simulink model "SPHERE_model4_PID_screenshot"  (R2020a)
settings: Solver=ode4  StartTime=0.0  StopTime=100  FixedStep=0.01428571  RelTol=1e-3
values from neighbouring files (symbols this model uses):
  Final_val = 18    [Initial_script.m]    (also in Initial_script_test.m = -28; Initial_script_test2.m = -28)
  K = 25.937    [Initial_script.m]    (also in Initial_script_test.m; Initial_script_test2.m)
  L = -[ M2*l*(-2*l + R) - 2*J2, 0, -2*M2*l*g ]    [Initial_script.m]    (also in Initial_script_test.m; Initial_script_test2.m)
  M = [ J1 + 2*J2 + M1*R^2 + M2*(2*l^2 - 3*R*l + R^2), -Tv, 2*l*g*M2 ]    [Initial_script.m]    (also in Initial_script_test.m; Initial_script_test2.m)
  Smax = 502    [Initial_script.m]    (also in Initial_script_test.m; Initial_script_test2.m)
  Smin = -480    [Initial_script.m]    (also in Initial_script_test.m; Initial_script_test2.m)
  Step_time = 3.18    [Initial_script.m]    (also in Initial_script_test.m = 4.45; Initial_script_test2.m = 4.5)
  Top = 0.015    [Initial_script.m]    (also in Initial_script_test.m; Initial_script_test2.m)
libraries: simulink x2
settings Model: Creator=Adrian  LastModifiedBy=Adrian

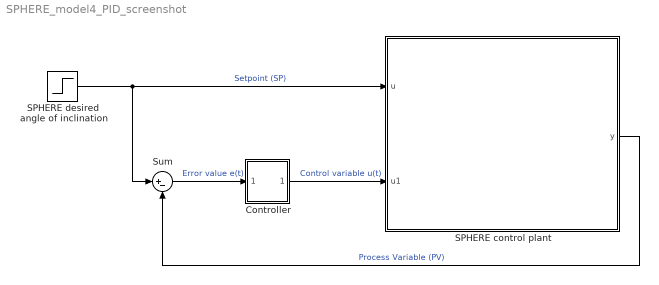
== system SPHERE_model4_PID_screenshot ==
  Controller : Subsystem  mask{Parameter1=}
      mask prompts: Parameter1 "Controller"
  SPHERE control plant : Subsystem
      mask Display: image('C:\Users\Adrian\Documents\Praca Magisterska\Robot kulisty by Adrian\Praca Magisterska\LaTex\Pictures\Old\sphere_full.PNG'); % Use "Edit Image" on toolstrip to change.
  SPHERE desired angle of inclination : Step  Time=Step_time  After=Final_val  SampleTime=0
  Sum : Sum  Inputs=|+-
  wires:
  SPHERE control plant/1(y) -> Sum/2  "Process Variable (PV)"
  SPHERE desired angle of inclination/1 -> Sum/1, SPHERE control plant/1(u)  "Setpoint (SP)"
  Sum/1 -> Controller/1(In1)  "Error value e(t)"
  Controller/1(Out1) -> SPHERE control plant/2(u1)  "Control variable u(t)"

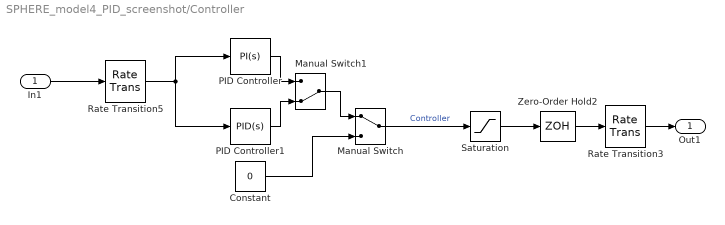
== system SPHERE_model4_PID_screenshot/Controller ==
  In1 : Inport
  Constant : Constant  Value=0
  Manual Switch : ManualSwitch
  Manual Switch1 : ManualSwitch  CurrentSetting=0
  PID Controller : simulink/Continuous/PID Controller  Controller=PI  Form=Parallel  TimeDomain=Continuous-time  UseExternalTs=off  SampleTime=-1  IntegratorMethod=Forward Euler  FilterMethod=Forward Euler  ControllerParametersSource=internal  P=-0.89  I=0.02  D=0  UseFilter=on  N=100  TunerSelectOption=Transfer Function Based (PID Tuner App)  InitialConditionSource=internal  InitialConditionForIntegrator=0  InitialConditionForFilter=0  DifferentiatorICPrevScaledInput=0  ExternalReset=none  TrackingMode=off  Kt=1  LimitOutput=off  UpperSaturationLimit=inf  LowerSaturationLimit=-inf  LinearizeAsGain=on  AntiWindupMode=none  Kb=1  POutMin=[]  POutMax=[]  IOutMin=[]  IOutMax=[]  DOutMin=[]  DOutMax=[]  NOutMin=[]  NOutMax=[]  SumOutMin=[]  SumOutMax=[]  SaturationOutMin=[]  SaturationOutMax=[]  PParamMin=[]  PParamMax=[]  IParamMin=[]  IParamMax=[]  DParamMin=[]  DParamMax=[]  NParamMin=[]  NParamMax=[]  KbParamMin=[]  KbParamMax=[]  KtParamMin=[]  KtParamMax=[]  KbOutMin=[]  KbOutMax=[]  KtOutMin=[]  KtOutMax=[]  IntegratorOutMin=[]  IntegratorOutMax=[]  FilterOutMin=[]  FilterOutMax=[]  SumI1OutMin=[]  SumI1OutMax=[]  SumI2OutMin=[]  SumI2OutMax=[]  SumI3OutMin=[]  SumI3OutMax=[]  SumI4OutMin=[]  SumI4OutMax=[]  SumDOutMin=[]  SumDOutMax=[]  DifferentiatorOutMin=[]  DifferentiatorOutMax=[]  FilterDiffOutCoefMin=[]  FilterDiffOutCoefMax=[]  ReciprocalOutMin=[]  ReciprocalOutMax=[]  SumDenOutMin=[]  SumDenOutMax=[]  SumNumOutMin=[]  SumNumOutMax=[]  DivideOutMin=[]  DivideOutMax=[]  UdiffTsProdOutMin=[]  UdiffTsProdOutMax=[]  NTsProdOutMin=[]  NTsProdOutMax=[]  UintegralTsProdOutMin=[]  UintegralTsProdOutMax=[]  UngainTsProdOutMin=[]  UngainTsProdOutMax=[]  IntegratorContinuousStateAttributes=''  IntegratorStateMustResolveToSignalObject=off  IntegratorRTWStateStorageClass=Auto  FilterContinuousStateAttributes=''  FilterStateMustResolveToSignalObject=off  FilterRTWStateStorageClass=Auto  ParallelPVariant=InternalParameters  IdealPVariant=Disabled  IVariant=InternalParameters  DVariant=Disabled  IntegratorVariant=Continuous  SatVariant=Disabled  AWVariant=Passthrough  PCopyVariant=Disabled  TRVariant=Disabled  FdbkBlocksVariant=Forward  IdealPFdbkVariant=Disabled  SatFdbkVariant=Disabled  DerivativeFilterVariant=Disabled  NVariant=Disabled  NCopyVariant=Disabled_SignalSpec  FilterICVariant=Disabled  IntegratorICVariant=InternalICs  ExternalResetVariant=Disabled  TRSumVariant=Passthrough  SumFdbkVariant=Disabled  SumVariant=Sum_PI  TsampFilterVariant=InternalTs  TsampNgainVariant=Passthrough  TsampIntegralVariant=Passthrough
  PID Controller1 : simulink/Continuous/PID Controller  Controller=PID  Form=Parallel  TimeDomain=Continuous-time  UseExternalTs=off  SampleTime=-1  IntegratorMethod=Forward Euler  FilterMethod=Forward Euler  ControllerParametersSource=internal  P=-0.9  I=0.035  D=0.07  UseFilter=on  N=100  TunerSelectOption=Transfer Function Based (PID Tuner App)  InitialConditionSource=internal  InitialConditionForIntegrator=0  InitialConditionForFilter=0  DifferentiatorICPrevScaledInput=0  ExternalReset=none  TrackingMode=off  Kt=1  LimitOutput=off  UpperSaturationLimit=inf  LowerSaturationLimit=-inf  LinearizeAsGain=on  AntiWindupMode=none  Kb=1  POutMin=[]  POutMax=[]  IOutMin=[]  IOutMax=[]  DOutMin=[]  DOutMax=[]  NOutMin=[]  NOutMax=[]  SumOutMin=[]  SumOutMax=[]  SaturationOutMin=[]  SaturationOutMax=[]  PParamMin=[]  PParamMax=[]  IParamMin=[]  IParamMax=[]  DParamMin=[]  DParamMax=[]  NParamMin=[]  NParamMax=[]  KbParamMin=[]  KbParamMax=[]  KtParamMin=[]  KtParamMax=[]  KbOutMin=[]  KbOutMax=[]  KtOutMin=[]  KtOutMax=[]  IntegratorOutMin=[]  IntegratorOutMax=[]  FilterOutMin=[]  FilterOutMax=[]  SumI1OutMin=[]  SumI1OutMax=[]  SumI2OutMin=[]  SumI2OutMax=[]  SumI3OutMin=[]  SumI3OutMax=[]  SumI4OutMin=[]  SumI4OutMax=[]  SumDOutMin=[]  SumDOutMax=[]  DifferentiatorOutMin=[]  DifferentiatorOutMax=[]  FilterDiffOutCoefMin=[]  FilterDiffOutCoefMax=[]  ReciprocalOutMin=[]  ReciprocalOutMax=[]  SumDenOutMin=[]  SumDenOutMax=[]  SumNumOutMin=[]  SumNumOutMax=[]  DivideOutMin=[]  DivideOutMax=[]  UdiffTsProdOutMin=[]  UdiffTsProdOutMax=[]  NTsProdOutMin=[]  NTsProdOutMax=[]  UintegralTsProdOutMin=[]  UintegralTsProdOutMax=[]  UngainTsProdOutMin=[]  UngainTsProdOutMax=[]  IntegratorContinuousStateAttributes=''  IntegratorStateMustResolveToSignalObject=off  IntegratorRTWStateStorageClass=Auto  FilterContinuousStateAttributes=''  FilterStateMustResolveToSignalObject=off  FilterRTWStateStorageClass=Auto  ParallelPVariant=InternalParameters  IdealPVariant=Disabled  IVariant=InternalParameters  DVariant=InternalParameters  IntegratorVariant=Continuous  SatVariant=Disabled  AWVariant=Passthrough  PCopyVariant=Disabled  TRVariant=Disabled  FdbkBlocksVariant=Forward  IdealPFdbkVariant=Disabled  SatFdbkVariant=Disabled  DerivativeFilterVariant=ContFilter  NVariant=InternalParameters  NCopyVariant=Disabled  FilterICVariant=InternalICsFilter  IntegratorICVariant=InternalICs  ExternalResetVariant=Disabled  TRSumVariant=Passthrough  SumFdbkVariant=Disabled  SumVariant=Sum_PID  TsampFilterVariant=InternalTs  TsampNgainVariant=Passthrough  TsampIntegralVariant=Passthrough
  Rate Transition3 : RateTransition
  Rate Transition5 : RateTransition
  Saturation : Saturate  UpperLimit=60  LowerLimit=-60
  Zero-Order Hold2 : ZeroOrderHold  SampleTime=-1
  Out1 : Outport
  wires:
  Constant/1 -> Manual Switch/2
  PID Controller/1 -> Manual Switch1/1
  Manual Switch/1 -> Saturation/1  "Controller"
  Zero-Order Hold2/1 -> Rate Transition3/1
  Manual Switch1/1 -> Manual Switch/1
  Rate Transition5/1 -> PID Controller1/1, PID Controller/1
  Rate Transition3/1 -> Out1/1
  Saturation/1 -> Zero-Order Hold2/1
  PID Controller1/1 -> Manual Switch1/2
  In1/1 -> Rate Transition5/1

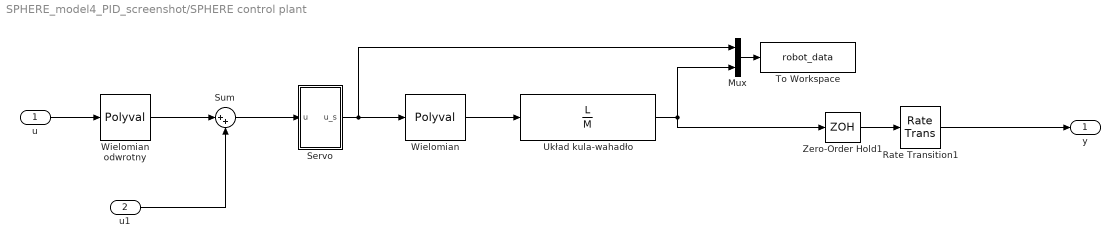
== system SPHERE_model4_PID_screenshot/SPHERE control plant ==
  u : Inport
  u1 : Inport  Port=2
  Mux : Mux  Inputs=2
  Rate Transition1 : RateTransition
  Servo : Subsystem
  Sum : Sum  Inputs=|++
  To Workspace : ToWorkspace  VariableName=robot_data  SaveFormat=Structure With Time  SampleTime=-1
  Układ kula-wahadło : TransferFcn  Numerator=L  Denominator=M
  Wielomian : Polyval  Coefs=[-0.000067 -0.000287 0.871698 0]
  Wielomian odwrotny : Polyval  Coefs=[0.000325 0.001274 1.044515 0]
  Zero-Order Hold1 : ZeroOrderHold  SampleTime=-1
  y : Outport
  wires:
  Układ kula-wahadło/1 -> Mux/2, Zero-Order Hold1/1
  Servo/1(u_s) -> Wielomian/1, Mux/1
  Mux/1 -> To Workspace/1
  Zero-Order Hold1/1 -> Rate Transition1/1
  Rate Transition1/1 -> y/1
  Wielomian/1 -> Układ kula-wahadło/1
  Sum/1 -> Servo/1(u)
  Wielomian odwrotny/1 -> Sum/1
  u1/1 -> Sum/2
  u/1 -> Wielomian odwrotny/1

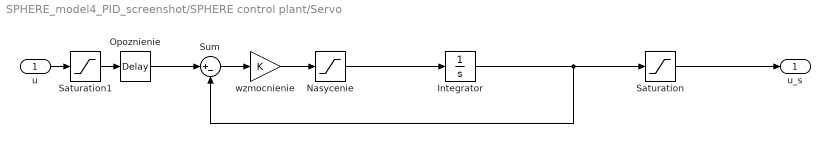
== system SPHERE_model4_PID_screenshot/SPHERE control plant/Servo ==
  u : Inport
  Integrator : Integrator
  Nasycenie : Saturate  UpperLimit=Smax  LowerLimit=Smin
  Opoznienie : TransportDelay  DelayTime=Top
  Saturation : Saturate  UpperLimit=60  LowerLimit=-60
  Saturation1 : Saturate  UpperLimit=60  LowerLimit=-60
  Sum : Sum  Inputs=|+-
  wzmocnienie : Gain  Gain=K
  u_s : Outport
  wires:
  Sum/1 -> wzmocnienie/1
  Integrator/1 -> Saturation/1, Sum/2
  wzmocnienie/1 -> Nasycenie/1
  Opoznienie/1 -> Sum/1
  Nasycenie/1 -> Integrator/1
  u/1 -> Saturation1/1
  Saturation/1 -> u_s/1
  Saturation1/1 -> Opoznienie/1
